simulink model "scenario3"  (Simulink 9.1)
settings: Solver=VariableStepAuto  StartTime=0.0  StopTime=30  RelTol=1e-3
undefined symbols (not defined in the file or in its folder): sigbuilder_block
libraries: fuzblock x1, simulink x1
settings Model: LogicAnalyzerSignalOrdering=3b64b31e-d3cb-4f80-974a-acfb4a65f103,3c1c965d-d39a-4847-8381-73e7e31213b0,712135b9-c1a7-43b3-afb3-76a269b195b3,9deb542a-15d4-4c32-b663-8057bef54c09  Creator=Dimitris  LastModifiedBy=Dimitris
settings DataIOCC: SaveFormat=Dataset
settings OptimizationCC: LifeSpan=auto
settings DebuggingCC: UnderspecifiedInitializationDetection=Simplified  MergeDetectMultiDrivingBlocksExec=error  SFUnexpectedBacktrackingDiag=error  SFNoUnconditionalDefaultTransitionDiag=error  SFExecutionAtInitializationDiag=warning
settings HardwareCC: ProdBitPerPointer=64  ProdBitPerSizeT=64  ProdBitPerPtrDiffT=64  ProdLargestAtomicFloat=Float  ProdIntDivRoundTo=Zero  ProdEndianess=LittleEndian  ProdWordSize=64  ProdHWDeviceType=Intel->x86-64 (Windows64)
settings ModelReferenceCC: PropagateSignalLabelsOutOfModel=on
settings CodeAppCC: StateflowObjectComments=off
settings GRTTargetCC: TargetLangStandard=C99 (ISO)  CombineOutputUpdateFcns=on  GRTInterface=off
settings ConfigComp: CovMetricSettings=dwe  CovHtmlReporting=off  CovSaveCumulativeToWorkspaceVar=off  CovSaveSingleToWorkspaceVar=off  CovExternalEMLEnable=on

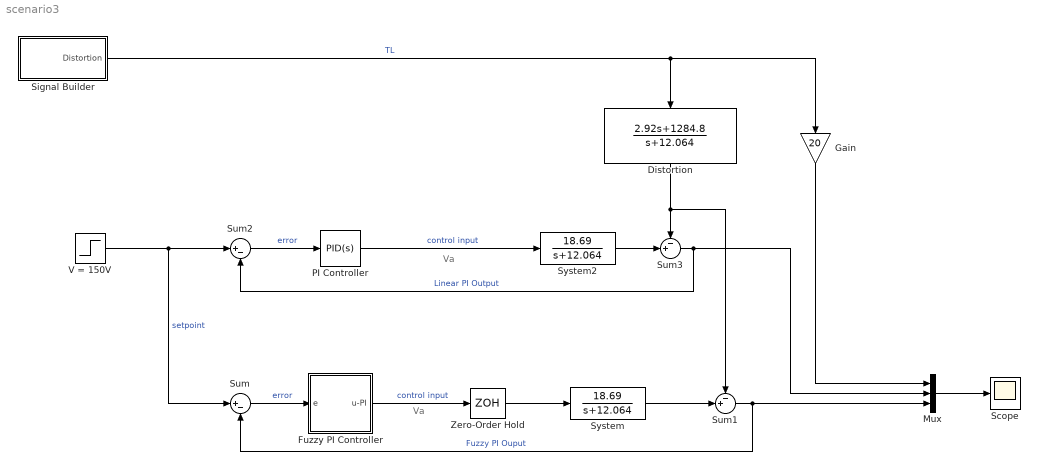
== system scenario3 ==
  note: Va
  note: Va
  Distortion : TransferFcn  Numerator=[2.92 1284.8]  Denominator=[1 12.064]
  Fuzzy PI Controller : Subsystem
  Gain : Gain  Gain=20
  Mux : Mux  Inputs=3
  PI Controller : simulink/Continuous/PID Controller  Controller=PID  TimeDomain=Continuous-time  SampleTime=-1  IntegratorMethod=Forward Euler  FilterMethod=Forward Euler  Form=Parallel  UseFilter=on  ControllerParametersSource=internal  P=1  I=1  D=0  N=100  InitialConditionSource=internal  InitialConditionForIntegrator=0  InitialConditionForFilter=0  ExternalReset=none  LimitOutput=off  UpperSaturationLimit=inf  LowerSaturationLimit=-inf  LinearizeAsGain=on  AntiWindupMode=none  Kb=1  TrackingMode=off  Kt=1  PParamMin=[]  PParamMax=[]  IParamMin=[]  IParamMax=[]  DParamMin=[]  DParamMax=[]  NParamMin=[]  NParamMax=[]  KbParamMin=[]  KbParamMax=[]  KtParamMin=[]  KtParamMax=[]  POutMin=[]  POutMax=[]  IOutMin=[]  IOutMax=[]  DOutMin=[]  DOutMax=[]  NOutMin=[]  NOutMax=[]  KbOutMin=[]  KbOutMax=[]  KtOutMin=[]  KtOutMax=[]  IntegratorOutMin=[]  IntegratorOutMax=[]  FilterOutMin=[]  FilterOutMax=[]  SumOutMin=[]  SumOutMax=[]  SumI1OutMin=[]  SumI1OutMax=[]  SumI2OutMin=[]  SumI2OutMax=[]  SumI3OutMin=[]  SumI3OutMax=[]  SumDOutMin=[]  SumDOutMax=[]  SaturationOutMin=[]  SaturationOutMax=[]  IntegratorContinuousStateAttributes=''  IntegratorStateMustResolveToSignalObject=off  IntegratorRTWStateStorageClass=Auto  FilterContinuousStateAttributes=''  FilterStateMustResolveToSignalObject=off  FilterRTWStateStorageClass=Auto  DifferentiatorICPrevScaledInput=0  DifferentiatorOutMin=[]  DifferentiatorOutMax=[]  FilterDiffOutCoefMin=[]  FilterDiffOutCoefMax=[]  SumDenOutMin=[]  SumDenOutMax=[]  SumNumOutMin=[]  SumNumOutMax=[]  ReciprocalOutMin=[]  ReciprocalOutMax=[]  DivideOutMin=[]  DivideOutMax=[]  TunerSelectOption=Transfer Function Based (PID Tuner App)
  Scope : Scope
  Signal Builder : Subsystem  Tag=STV Subsys  LoadFcn=sigbuilder_block('load');  StartFcn=sigbuilder_block('start');  StopFcn=sigbuilder_block('stop');  ClipboardFcn=sigbuilder_block('clipboard');  mask(Sigbuilder block){tuvar=[0:10]}
      mask help: Simulink:masks:SigbuilderBlock_MD
      mask init:
      | if ~strcmp(get_param(bdroot(gcbh),'SimulationStatus'),'stopped') tuvar = sigbuilder_block('maskInit'); end
      settings: CopyFcn=sigbuilder_block('copy');  DeleteFcn=sigbuilder_block('delete');  ModelCloseFcn=sigbuilder_block('modelClose');  PreSaveFcn=sigbuilder_block('preSave');  PauseFcn=sigbuilder_block('pause');  ContinueFcn=sigbuilder_block('continue');  NameChangeFcn=sigbuilder_block('namechange');  OpenFcn=sigbuilder_block('open',[437.6 199.2 550.4 400 ]);  CloseFcn=sigbuilder_block('close');
      mask Display: plot(0, 0, 100, 100,[2, 2, 32, 32, 2], [68, 8, 8, 68, 68],[32, 2], [38, 38], [32, 19, 2],[53, 60, 44], [32, 17, 17, 2],[16, 16, 31, 31]);txt = getActiveGroup(gcbh);text(2, 100, txt,'verticalAlignment', 'top');
  Sum : Sum  Inputs=|+-
  Sum1 : Sum  Inputs=-+|
  Sum2 : Sum  Inputs=|+-
  Sum3 : Sum  Inputs=-+|
  System : TransferFcn  Numerator=[18.69]  Denominator=[1 12.064]
  System2 : TransferFcn  Numerator=[18.69]  Denominator=[1 12.064]
  V = 150V : Step  Time=0  After=150  SampleTime=0
  Zero-Order Hold : ZeroOrderHold  SampleTime=0.01
  wires:
  Mux/1 -> Scope/1
  Sum/1 -> Fuzzy PI Controller/1(e)  "error"
  Zero-Order Hold/1 -> System/1
  Fuzzy PI Controller/1(u-PI) -> Zero-Order Hold/1  "control input"
  System/1 -> Sum1/2
  Signal Builder/1(Distortion) -> Distortion/1, Gain/1  "TL"
  Gain/1 -> Mux/1
  Sum2/1 -> PI Controller/1  "error"
  PI Controller/1 -> System2/1  "control input"
  System2/1 -> Sum3/2
  Distortion/1 -> Sum1/1, Sum3/1
  Sum3/1 -> Mux/2, Sum2/2  "Linear PI Output"
  V = 150V/1 -> Sum/1, Sum2/1  "setpoint"
  Sum1/1 -> Sum/2, Mux/3  "Fuzzy PI Ouput"

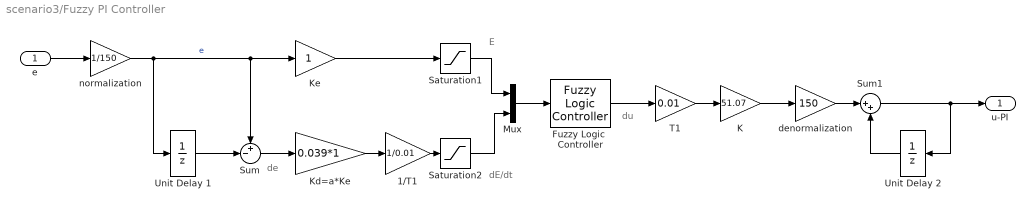
== system scenario3/Fuzzy PI Controller ==
  note: E
  note: de
  note: dE/dt
  note: du
  e : Inport
  1/T1 : Gain  Gain=1/0.01
  "Fuzzy Logic  Controller " : fuzblock/Fuzzy Logic  Controller  FIS='FIS_COA.fis'  OutputSampleNumber=101  DataType=double  FuzzifiedInputs=off  RuleFiringStrengths=off  RuleOutputs=off  AggregatedOutputs=off  SimulateUsing=Interpreted execution  OutOfRangeInputValueMessage=warning  NoRuleFiredMessage=warning  EmptyOutputFuzzySetMessage=warning
  K : Gain  Gain=51.07
  Kd=a*Ke : Gain  Gain=0.039*1
  Ke : Gain
  Mux : Mux  Inputs=2
  Saturation1 : Saturate  UpperLimit=1  LowerLimit=-1
  Saturation2 : Saturate  UpperLimit=1  LowerLimit=-1
  Sum : Sum  Inputs=+-|
  Sum1 : Sum  Inputs=|++
  "T1 " : Gain  Gain=0.01
  Unit Delay 1 : UnitDelay  SampleTime=0.01
  Unit Delay 2 : UnitDelay  SampleTime=0.01
  denormalization : Gain  Gain=150
  normalization : Gain  Gain=1/150
  u-PI : Outport
  wires:
  e/1 -> normalization/1
  normalization/1 -> Unit Delay 1/1, Sum/1, Ke/1  "e"
  Unit Delay 1/1 -> Sum/2
  Sum/1 -> Kd=a*Ke/1
  Kd=a*Ke/1 -> 1/T1/1
  Ke/1 -> Saturation1/1
  1/T1/1 -> Saturation2/1
  Saturation1/1 -> Mux/1
  Saturation2/1 -> Mux/2
  "T1 "/1 -> K/1
  K/1 -> denormalization/1
  denormalization/1 -> Sum1/1
  Sum1/1 -> u-PI/1, Unit Delay 2/1
  Unit Delay 2/1 -> Sum1/2
  "Fuzzy Logic  Controller "/1 -> "T1 "/1
  Mux/1 -> "Fuzzy Logic  Controller "/1

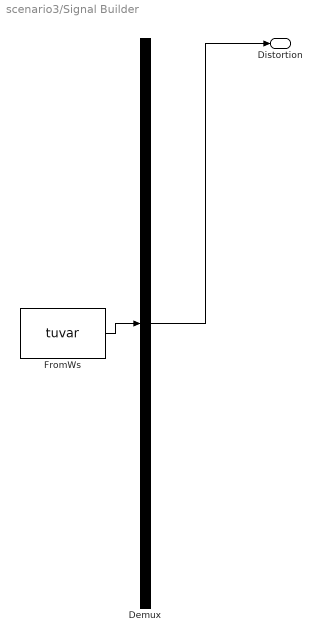
== system scenario3/Signal Builder ==
  Demux : Demux  Tag=STV Demux  Outputs=1
  FromWs : FromWorkspace  Tag=STV FromWs  VariableName=tuvar  SampleTime=0  SigBuilderData=DataTag0  VnvData=DataTag1
      SigBuilderData=|
      | common.afterFinalStr = 'Extrapolate'
      | common.sampleTime = 0
      | dataSet.timeRange = [0 30]
      | dataSet.name = 'TL'
      | sbobj.Groups.Name = 'TL'
      | sbobj.Groups.Signals.Name = 'Distortion'
      | sbobj.Groups.Signals.XData = [0 10 10 20 20.05 30]
      | sbobj.Groups.Signals.YData = [0 0 1 1 0 0]
      | sbobj.Groups.TimeRange = [0 30]
  Distortion : Outport  Tag=STV Outport
  wires:
  Demux/1 -> Distortion/1
  FromWs/1 -> Demux/1
